simulink model "rendezvous_optimization_WOA"  (R2023a)
settings: Solver=VariableStepAuto  StartTime=0.0  StopTime=100  RelTol=1e-3
values from neighbouring files (symbols this model uses):
  Ax = [0,1;(3*(omega_T^2)),0]    [position_control.m]    (also in satellite_model.m)
  Ax_i = [0,1;0,0]    [position_control.m]    (also in satellite_model.m)
  Ay = [0,1;0,0]    [position_control.m]    (also in satellite_model.m)
  Ay_i = [0,1;0,0]    [position_control.m]    (also in satellite_model.m)
  Az = [0,1;(-(omega_T^2)),0]    [position_control.m]    (also in satellite_model.m)
  Bx = [0;1/m0]    [position_control.m]    (also in satellite_model.m)
  Bx_i = [0;1/m0]    [position_control.m]    (also in satellite_model.m)
  By = [0;1/m0]    [position_control.m]    (also in satellite_model.m)
  By_i = [0;1/m0]    [position_control.m]    (also in satellite_model.m)
  Bz = [0;1/m0]    [position_control.m]    (also in satellite_model.m)
  Cx = eye(2)    [position_control.m]    (also in satellite_model.m)
  Cx_i = eye(2)    [position_control.m]    (also in satellite_model.m)
  Cy = eye(2)    [position_control.m]    (also in satellite_model.m)
  Cy_i = eye(2)    [position_control.m]    (also in satellite_model.m)
  Cz = eye(2)    [position_control.m]    (also in satellite_model.m)
  IC_x_init = [icrf_pos_x(1);icrf_vel_x(1)]    [position_control.m]
  IC_y_init = [icrf_pos_y(2);icrf_vel_y(2)]    [position_control.m]
  m0 = 4    [position_control.m]    (also in satellite_model.m)
  mDot = 0.000102    [position_control.m]    (also in satellite_model.m)
  OC_x_init = [hill_pos_x(1);hill_vel_x(1)]    [position_control.m]
  OC_y_init = [hill_pos_y(2);hill_vel_y(2)]    [position_control.m]
  OC_z_init = [hill_pos_z(3);hill_vel_z(3)]    [position_control.m]
  omega_T = deg2rad(0.1)    [position_control.m]    (also in satellite_model.m)
  Ve = [Ve_x; 0; 0]    [position_control.m]    (also in satellite_model.m)
undefined symbols (not defined in the file or in its folder): juliandate
(part 2 of 2)

== matlab function rendezvous_optimization_WOA/Deputy Spacecraft/Guidance and Control/Control/Translational Controller/Outer Controller-y/Controller-2/MATLAB Function ==
  settings: updateMethod=DISCRETE
  data: bestKi output; bestKp output; bestKd output; error input
function [bestKi,bestKp,bestKd] = whale(error)
%% WOA_PID_Tuning.m
%----------------------------------------------------------------------
% Whale Optimization Algorithm for PID Tuning

%% 2) WOA parameters
nWhales  = 100;                % population size
Max_iter = 100;               % number of iterations
lb       = [0   0   0];       % [Kp_min, Ki_min, Kd_min]
ub       = [30  20  30];       % [Kp_max, Ki_max, Kd_max]

%% 3) Run WOA
bestGains = runWOA(error, nWhales, Max_iter, lb, ub);
bestKp = bestGains(1);
bestKi = bestGains(2);
bestKd = bestGains(3);

%======================================================================
% runWOA: core Whale Optimization Algorithm
%======================================================================
function bestGains = runWOA(error, nWhales, Max_iter, lb, ub)
    dim = numel(lb);                      % 3 gains to tune
    whales   = rand(nWhales,dim).*(ub-lb) + lb;  % initialize
    fitness  = zeros(nWhales,1);
    
    % evaluate initial fitness
    for i = 1:nWhales
        fitness(i) = error;
    end
    [bestFit, idx] = min(fitness);
    bestWhale      = whales(idx,:);

    b = 1;  % spiral parameter

    for iter = 1:Max_iter
        a = 2*(1 - iter/Max_iter);  % linearly decreases from 2 to 0

        for i = 1:nWhales
            r = rand;                 C = 2*rand;
            A = 2*a*r - a;            % coefficient for exploitation/exploration
            p = rand;

            if p < 0.5
                if abs(A) < 1
                    % Encircling the best solution
                    D = abs(C*bestWhale - whales(i,:));
                    whales(i,:) = bestWhale - A.*D;
                else
                    % Exploration: encircle a random whale
                    randIdx = randi(nWhales);
                    X_rand  = whales(randIdx,:);
                    D       = abs(C*X_rand - whales(i,:));
                    whales(i,:) = X_rand - A.*D;
                end
            else
                % Bubble-net spiral (exploitation)
                D = abs(bestWhale - whales(i,:));
                l = -1 + 2*rand;  % random in [−1,1]
                whales(i,:) = D.*exp(b*l).*cos(2*pi*l) + bestWhale;
            end

            % enforce bounds
            whales(i,:) = max(min(whales(i,:), ub), lb);
        end

        % re‐evaluate fitness
        for i = 1:nWhales
            fitness(i) = error;
        end
        [currBest, idx] = min(fitness);
        if currBest < bestFit
            bestFit    = currBest;
            bestWhale  = whales(idx,:);
        end
    end

    bestGains = bestWhale;
end

  
end

== matlab function rendezvous_optimization_WOA/Deputy Spacecraft/Guidance and Control/Control/Translational Controller/Outer Controller-z/Controller-3/MATLAB Function ==
  settings: updateMethod=DISCRETE
  data: bestKi output; bestKp output; bestKd output; error input
function [bestKi,bestKp,bestKd] = whale(error)
%% WOA_PID_Tuning.m
%----------------------------------------------------------------------
% Whale Optimization Algorithm for PID Tuning

%% 2) WOA parameters
nWhales  = 100;                % population size
Max_iter = 100;               % number of iterations
lb       = [0   0   0];       % [Kp_min, Ki_min, Kd_min]
ub       = [30  20  30];       % [Kp_max, Ki_max, Kd_max]

%% 3) Run WOA
bestGains = runWOA(error, nWhales, Max_iter, lb, ub);
bestKp = bestGains(1);
bestKi = bestGains(2);
bestKd = bestGains(3);


%======================================================================
% runWOA: core Whale Optimization Algorithm
%======================================================================
function bestGains = runWOA(error, nWhales, Max_iter, lb, ub)
    dim = numel(lb);                      % 3 gains to tune
    whales   = rand(nWhales,dim).*(ub-lb) + lb;  % initialize
    fitness  = zeros(nWhales,1);
    
    % evaluate initial fitness
    for i = 1:nWhales
        fitness(i) = error;
    end
    [bestFit, idx] = min(fitness);
    bestWhale      = whales(idx,:);

    b = 1;  % spiral parameter

    for iter = 1:Max_iter
        a = 2*(1 - iter/Max_iter);  % linearly decreases from 2 to 0

        for i = 1:nWhales
            r = rand;                 C = 2*rand;
            A = 2*a*r - a;            % coefficient for exploitation/exploration
            p = rand;

            if p < 0.5
                if abs(A) < 1
                    % Encircling the best solution
                    D = abs(C*bestWhale - whales(i,:));
                    whales(i,:) = bestWhale - A.*D;
                else
                    % Exploration: encircle a random whale
                    randIdx = randi(nWhales);
                    X_rand  = whales(randIdx,:);
                    D       = abs(C*X_rand - whales(i,:));
                    whales(i,:) = X_rand - A.*D;
                end
            else
                % Bubble-net spiral (exploitation)
                D = abs(bestWhale - whales(i,:));
                l = -1 + 2*rand;  % random in [−1,1]
                whales(i,:) = D.*exp(b*l).*cos(2*pi*l) + bestWhale;
            end

            % enforce bounds
            whales(i,:) = max(min(whales(i,:), ub), lb);
        end

        % re‐evaluate fitness
        for i = 1:nWhales
            fitness(i) = error;
        end
        [currBest, idx] = min(fitness);
        if currBest < bestFit
            bestFit    = currBest;
            bestWhale  = whales(idx,:);
        end
    end

    bestGains = bestWhale;
end

  
end

== matlab function rendezvous_optimization_WOA/Deputy Spacecraft/Guidance and Control/Control/Translational Controller/Inner Controller-x/Subsystem/MATLAB Function ==
  settings: updateMethod=DISCRETE
  data: bestKi output; bestKp output; bestKd output; error input
function [bestKi,bestKp,bestKd] = whale(error)
%% WOA_PID_Tuning.m
%----------------------------------------------------------------------
% Whale Optimization Algorithm for PID Tuning

%% 2) WOA parameters
nWhales  = 100;                % population size
Max_iter = 100;               % number of iterations
lb       = [0   0   0];       % [Kp_min, Ki_min, Kd_min]
ub       = [10  5  10];       % [Kp_max, Ki_max, Kd_max]

%% 3) Run WOA
bestGains = runWOA(error, nWhales, Max_iter, lb, ub);
bestKp = bestGains(1);
bestKi = bestGains(2);
bestKd = bestGains(3);

%======================================================================
% runWOA: core Whale Optimization Algorithm
%======================================================================
function bestGains = runWOA(error, nWhales, Max_iter, lb, ub)
    dim = numel(lb);                      % 3 gains to tune
    whales   = rand(nWhales,dim).*(ub-lb) + lb;  % initialize
    fitness  = zeros(nWhales,1);
    
    % evaluate initial fitness
    for i = 1:nWhales
        fitness(i) = error;
    end
    [bestFit, idx] = min(fitness);
    bestWhale      = whales(idx,:);

    b = 1;  % spiral parameter

    for iter = 1:Max_iter
        a = 2*(1 - iter/Max_iter);  % linearly decreases from 2 to 0

        for i = 1:nWhales
            r = rand;                 C = 2*rand;
            A = 2*a*r - a;            % coefficient for exploitation/exploration
            p = rand;

            if p < 0.5
                if abs(A) < 1
                    % Encircling the best solution
                    D = abs(C*bestWhale - whales(i,:));
                    whales(i,:) = bestWhale - A.*D;
                else
                    % Exploration: encircle a random whale
                    randIdx = randi(nWhales);
                    X_rand  = whales(randIdx,:);
                    D       = abs(C*X_rand - whales(i,:));
                    whales(i,:) = X_rand - A.*D;
                end
            else
                % Bubble-net spiral (exploitation)
                D = abs(bestWhale - whales(i,:));
                l = -1 + 2*rand;  % random in [−1,1]
                whales(i,:) = D.*exp(b*l).*cos(2*pi*l) + bestWhale;
            end

            % enforce bounds
            whales(i,:) = max(min(whales(i,:), ub), lb);
        end

        % re‐evaluate fitness
        for i = 1:nWhales
            fitness(i) = error;
        end
        [currBest, idx] = min(fitness);
        if currBest < bestFit
            bestFit    = currBest;
            bestWhale  = whales(idx,:);
        end
    end

    bestGains = bestWhale;
end

  
end

== matlab function rendezvous_optimization_WOA/Deputy Spacecraft/Guidance and Control/Control/Translational Controller/Outer Controller-x/Controller-1/MATLAB Function1 ==
  settings: updateMethod=DISCRETE
  data: reset input; error_percent output; error input
function error_percent = computeScheduledGain(reset,error)
% Compute gain based on percentage error using 1D look-up style logic
%
% Inputs:
%   r_des     : 3x1 desired position vector
%   r_current : 3x1 current position vector (from chaser)
%   r_init    : 3x1 initial position vector
%
% Output:
%   gain      : scalar scheduled gain

    persistent max_error;

    if reset || isempty(max_error)
        max_error = norm(error);  % store initial max error
    end
    
    e_now = norm(error);       % current error
    error_percent = (e_now / max_error)*100;       % normalized error: [0, 1]

   
end
